simulink model "test_basic"  (R2020b)
settings: Solver=VariableStepAuto  StartTime=0.0  StopTime=10.0  RelTol=1e-3
undefined symbols (not defined in the file): mergepose
libraries: simlib_vpc_basic x9, simlib_vpc_coremath x2
settings Model: Creator=marco  LastModifiedBy=marco

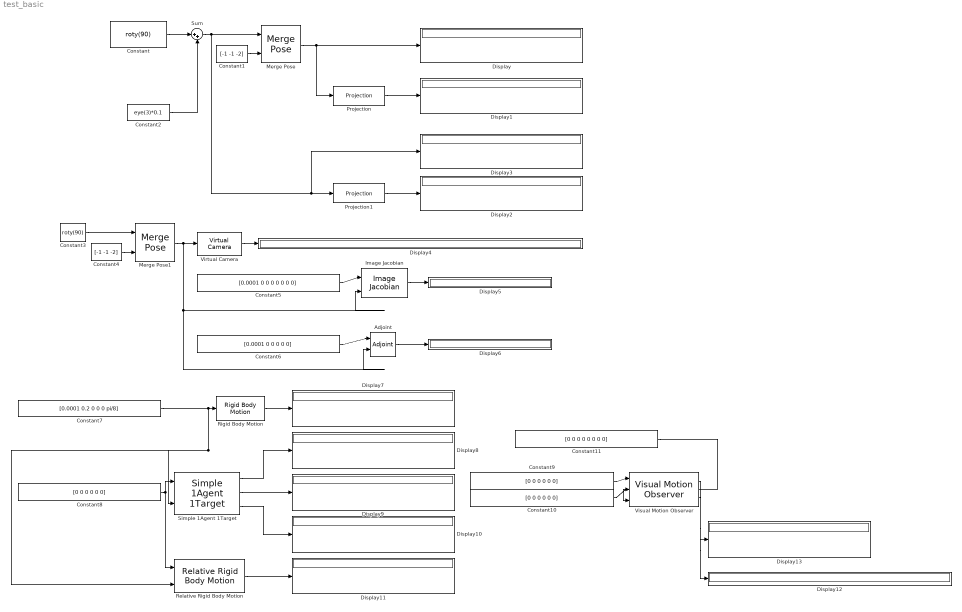
== system test_basic ==
  Adjoint : simlib_vpc_basic/Adjoint  adjointtype=pose
  Constant : Constant  Value=roty(90)
  Constant1 : Constant  Value=[-1 -1 -2]
  Constant10 : Constant  Value=[0 0 0 0 0 0]
  Constant11 : Constant  Value=[0 0 0 0 0 0 0 0]
  Constant2 : Constant  Value=eye(3)*0.1
  Constant3 : Constant  Value=roty(90)
  Constant4 : Constant  Value=[-1 -1 -2]
  Constant5 : Constant  Value=[0.0001 0 0 0 0 0 0 0]
  Constant6 : Constant  Value=[0.0001 0 0 0 0 0]
  Constant7 : Constant  Value=[0.0001 0.2 0 0 0 pi/8]
  Constant8 : Constant  Value=[0 0 0 0 0 0]
  Constant9 : Constant  Value=[0 0 0 0 0 0]
  Display{,1..13} (14 alike) : Display
  Image Jacobian : simlib_vpc_basic/Image Jacobian  po=[0, 10*sqrt(3), 0;15, -5*sqrt(3), 0;-15, -5*sqrt(3), 0;0, 0, 10*sqrt(6)]./100  lambda=0.0041
  Merge Pose : simlib_vpc_coremath/Merge Pose
      settings: SourceProductName=VPC Library
  Merge Pose1 : simlib_vpc_coremath/Merge Pose
      settings: SourceProductName=VPC Library
  Projection : simlib_vpc_basic/Projection  projectiontype=averaging  inputtype=pose
  Projection1 : simlib_vpc_basic/Projection  projectiontype=averaging  inputtype=rotation matrix
  Relative Rigid Body Motion : simlib_vpc_basic/Relative Rigid Body Motion  gco0=eye(4)  projection=on
  Rigid Body Motion : simlib_vpc_basic/Rigid Body Motion  rbmtype=agent  agentnumber=1  projection=on  g0=eye(4)
  Simple 1Agent 1Target : simlib_vpc_basic/Simple 1Agent 1Target  gwc0=mergepose(rotx(90),ones(1,3))  projectionAgent=on  gwo0=eye(4)  projectionTarget=on  showgwc=on  showgwo=on
  Sum : Sum  Inputs=|++
  Virtual Camera : simlib_vpc_basic/Virtual Camera  camtype=Pinhole  po=[0, 10*sqrt(3), 0;15, -5*sqrt(3), 0;-15, -5*sqrt(3), 0;0, 0, 10*sqrt(6)]./100  lambda=0.0041
  Visual Motion Observer : simlib_vpc_basic/Visual Motion Observer  gcobar0=eye(4)  projection=on  camtype=Pinhole  fo=[0, 10*sqrt(3), 0;15, -5*sqrt(3), 0;-15, -5*sqrt(3), 0;0, 0, 10*sqrt(6)]./100  lambda=0.0041
  wires:
  Constant/1 -> Sum/1
  Constant1/1 -> Merge Pose/2
  Merge Pose/1 -> Projection/1, Display/1
  Projection/1 -> Display1/1
  Constant2/1 -> Sum/2
  Sum/1 -> Display3/1, Projection1/1, Merge Pose/1
  Projection1/1 -> Display2/1
  Constant3/1 -> Merge Pose1/1
  Constant4/1 -> Merge Pose1/2
  Merge Pose1/1 -> Adjoint/2, Image Jacobian/2, Virtual Camera/1
  Virtual Camera/1 -> Display4/1
  Constant5/1 -> Image Jacobian/1
  Image Jacobian/1 -> Display5/1
  Constant6/1 -> Adjoint/1
  Adjoint/1 -> Display6/1
  Constant7/1 -> Relative Rigid Body Motion/2, Simple 1Agent 1Target/2, Rigid Body Motion/1
  Rigid Body Motion/1 -> Display7/1
  Constant8/1 -> Relative Rigid Body Motion/1, Simple 1Agent 1Target/1
  Simple 1Agent 1Target/1 -> Display8/1
  Simple 1Agent 1Target/2 -> Display9/1
  Simple 1Agent 1Target/3 -> Display10/1
  Relative Rigid Body Motion/1 -> Display11/1
  Constant9/1 -> Visual Motion Observer/1
  Constant10/1 -> Visual Motion Observer/2
  Constant11/1 -> Visual Motion Observer/3
  Visual Motion Observer/2 -> Display13/1
  Visual Motion Observer/1 -> Display12/1
